simulink model "gm_HDL_pfc_gold_fi_vnl"  (R2024b)
settings: Solver=FixedStepDiscrete  StartTime=0.0  StopTime=.06  RelTol=1e-3
InitFcn:
  | fidelity_pfc_vals;
  | load('C:\Users\angro\Desktop\hil\pfc3ph\matlab\sim\sschdl\pfc_desktop\stateSpaceParameters.mat');
undefined symbols (not defined in the file or in its folder): a, b, c, DiscIntNeverNeededParam, fsw, Gs, s, stateSpaceParameters_1, t_ss, tsw
libraries: simulink x55, hdlmdlgenlib x26, hdlsllib x10, mcbcontrolslib x5, dspsrcs4 x3, slpidlib x2, hdlssclib x2, spsSVPWMGenerator2LevelLib x1, spsPLL3phLib x1
(part 3 of 4)

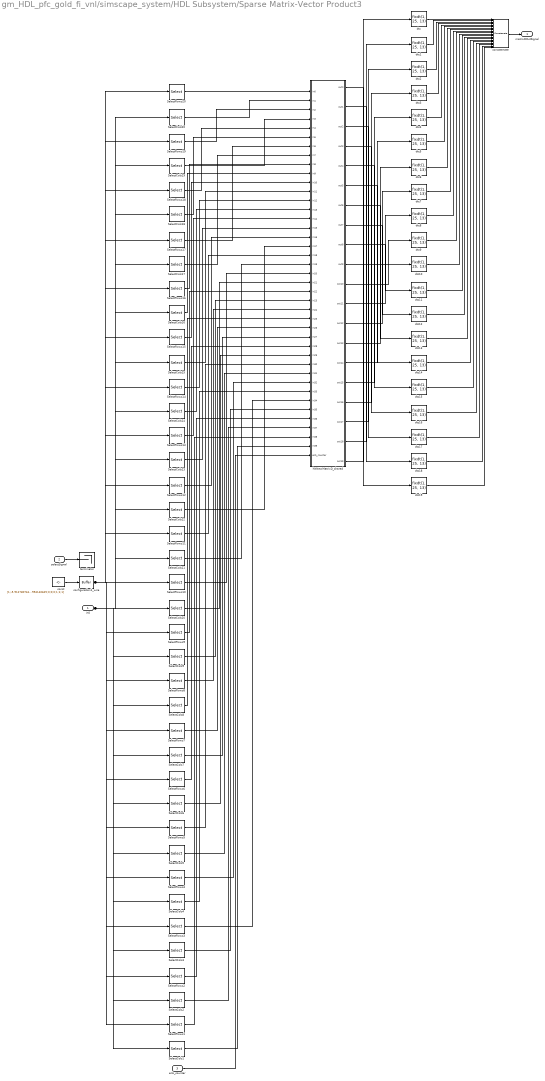
== system gm_HDL_pfc_gold_fi_vnl/simscape_system/HDL Subsystem/Sparse Matrix-Vector Product3 ==
  in0 : Inport  OutDataTypeStr=fixdt(1, 25, 13)  PortDimensions=[10]  SampleTime=1.38600138600139e-08
  selectSignal : Inport  Port=2  OutDataTypeStr=boolean  SampleTime=1.38600138600139e-08
  enb_counter : Inport  Port=3  OutDataTypeStr=fixdt(0, 6, 0)  SampleTime=1.38600138600139e-08
  SelectCols{1..17} (17 alike) : Selector  InputPortWidth=10  IndexOptions=Index vector (dialog)  Indices=double([1 2 3 4 5 6 7])  OutputSizes=double(1)
  SelectCols18 : Selector  InputPortWidth=10  IndexOptions=Index vector (dialog)  Indices=double([1 2 3 4 5 6 9])  OutputSizes=double(1)
  SelectCols19 : Selector  InputPortWidth=10  IndexOptions=Index vector (dialog)  Indices=double([1 2 3 4 5 6 10])  OutputSizes=double(1)
  SelectCols20 : Selector  InputPortWidth=10  IndexOptions=Index vector (dialog)  Indices=double([1 2 3 4 5 6 8])  OutputSizes=double(1)
  SelectRows1 : Selector  InputPortWidth=140  IndexOptions=Index vector (dialog)  Indices=double([1 21 41 61 81 101 121])  OutputSizes=double(1)
  SelectRows10 : Selector  InputPortWidth=140  IndexOptions=Index vector (dialog)  Indices=double([10 30 50 70 90 110 130])  OutputSizes=double(1)
  SelectRows11 : Selector  InputPortWidth=140  IndexOptions=Index vector (dialog)  Indices=double([11 31 51 71 91 111 131])  OutputSizes=double(1)
  SelectRows12 : Selector  InputPortWidth=140  IndexOptions=Index vector (dialog)  Indices=double([12 32 52 72 92 112 132])  OutputSizes=double(1)
  SelectRows13 : Selector  InputPortWidth=140  IndexOptions=Index vector (dialog)  Indices=double([13 33 53 73 93 113 133])  OutputSizes=double(1)
  SelectRows14 : Selector  InputPortWidth=140  IndexOptions=Index vector (dialog)  Indices=double([14 34 54 74 94 114 134])  OutputSizes=double(1)
  SelectRows15 : Selector  InputPortWidth=140  IndexOptions=Index vector (dialog)  Indices=double([15 35 55 75 95 115 135])  OutputSizes=double(1)
  SelectRows16 : Selector  InputPortWidth=140  IndexOptions=Index vector (dialog)  Indices=double([16 36 56 76 96 116 136])  OutputSizes=double(1)
  SelectRows17 : Selector  InputPortWidth=140  IndexOptions=Index vector (dialog)  Indices=double([17 37 57 77 97 117 137])  OutputSizes=double(1)
  SelectRows18 : Selector  InputPortWidth=140  IndexOptions=Index vector (dialog)  Indices=double([18 38 58 78 98 118 139])  OutputSizes=double(1)
  SelectRows19 : Selector  InputPortWidth=140  IndexOptions=Index vector (dialog)  Indices=double([19 39 59 79 99 119 140])  OutputSizes=double(1)
  SelectRows2 : Selector  InputPortWidth=140  IndexOptions=Index vector (dialog)  Indices=double([2 22 42 62 82 102 122])  OutputSizes=double(1)
  SelectRows20 : Selector  InputPortWidth=140  IndexOptions=Index vector (dialog)  Indices=double([20 40 60 80 100 120 138])  OutputSizes=double(1)
  SelectRows3 : Selector  InputPortWidth=140  IndexOptions=Index vector (dialog)  Indices=double([3 23 43 63 83 103 123])  OutputSizes=double(1)
  SelectRows4 : Selector  InputPortWidth=140  IndexOptions=Index vector (dialog)  Indices=double([4 24 44 64 84 104 124])  OutputSizes=double(1)
  SelectRows5 : Selector  InputPortWidth=140  IndexOptions=Index vector (dialog)  Indices=double([5 25 45 65 85 105 125])  OutputSizes=double(1)
  SelectRows6 : Selector  InputPortWidth=140  IndexOptions=Index vector (dialog)  Indices=double([6 26 46 66 86 106 126])  OutputSizes=double(1)
  SelectRows7 : Selector  InputPortWidth=140  IndexOptions=Index vector (dialog)  Indices=double([7 27 47 67 87 107 127])  OutputSizes=double(1)
  SelectRows8 : Selector  InputPortWidth=140  IndexOptions=Index vector (dialog)  Indices=double([8 28 48 68 88 108 128])  OutputSizes=double(1)
  SelectRows9 : Selector  InputPortWidth=140  IndexOptions=Index vector (dialog)  Indices=double([9 29 49 69 89 109 129])  OutputSizes=double(1)
  concatenate : Concatenate  NumInputs=20
  configuration1_wire : hdlmdlgenlib/Buffer
  const : Constant  Value=[1;-5.91278076171875e-05;-0.0030002593994140625;-5.91278076171875e-05;-0.0030002593994140625;-5.91278076171875e-05;-0.0030002593994140625;-5.91278076171875e-05;-0.0030002593994140625;-5.91278076171875e-05;-0.0030002593994140625;-5.91278076171875e-05;-0.0030002593994140625;-0.0059986114501953125;0;0;0;0;0;0;0;-0.499969482421875;25.001499176025390625;-0.499969482421875;-24.998500823974609375;3.0517578125e-05;0.001499176025390625;3.0517578125e-05;0.001499176025390625;3.0517578125e-05;0.001499176025390625;3.0517578125e-05;0.001499176025390625;0.0030002593994140625;0;0;0;0;0;0;0;-0.499969482421875;-24.998500823974609375;-0.499969482421875;25.001499176025390625;3.0517578125e-05;0.001499176025390625;3.0517578125e-05;0.001499176025390625;3.0517578125e-05;0.001499176025390625;3.0517578125e-05;0.001499176025390625;0.0030002593994140625;0;0;0;0;0;0;0;3.0517578125e-05;0.001499176025390625;3.0517578125e-05;0.001499176025390625;-0.499969482421875;25.001499176025390625;3.0517578125e-05;0.001499176025390625;-0.499969482421875;-24.998500823974609375;3.0517578125e-05;0.001499176025390625;0.0030002593994140625;0;0;0;0;0;0;0;3.0517578125e-05;0.001499176025390625;3.0517578125e-05;0.001499176025390625;3.0517578125e-05;0.001499176025390625;-0.499969482421875;25.001499176025390625;3.0517578125e-05;0.001499176025390625;-0.499969482421875;-24.998500823974609375;0.0030002593994140625;0;0;0;0;0;0;0;3.0517578125e-05;0.001499176025390625;3.0517578125e-05;0.001499176025390625;-0.499969482421875;-24.998500823974609375;3.0517578125e-05;0.001499176025390625;-0.499969482421875;25.001499176025390625;3.0517578125e-05;0.001499176025390625;0.0030002593994140625;0;0;0;0;0;0;0;3.0517578125e-05;0.001499176025390625;3.0517578125e-05;0.001499176025390625;3.0517578125e-05;0.001499176025390625;-0.499969482421875;-24.998500823974609375;3.0517578125e-05;0.001499176025390625;-0.499969482421875;25.001499176025390625;0.0030002593994140625;0;0;0;1;1;1]  OutDataTypeStr=fixdt(1, 25, 19)  SampleTime=1.38600138600139e-08
  dtc{,1..19} (20 alike) : DataTypeConversion  OutDataTypeStr=fixdt(1, 25, 13)  RndMeth=Nearest  SampleTime=1.38600138600139e-08  SaturateOnIntegerOverflow=off
  hNNewMatrixD_shared : Subsystem
  terminator : Terminator
  matrixDOutSignal : Outport  OutDataTypeStr=fixdt(1, 25, 13)  PortDimensions=[20]  SampleTime=1.38600138600139e-08
  wires:
  concatenate/1 -> matrixDOutSignal/1
  dtc19/1 -> concatenate/20
  dtc18/1 -> concatenate/19
  dtc17/1 -> concatenate/18
  dtc16/1 -> concatenate/17
  dtc15/1 -> concatenate/16
  dtc14/1 -> concatenate/15
  dtc13/1 -> concatenate/14
  dtc12/1 -> concatenate/13
  dtc11/1 -> concatenate/12
  dtc10/1 -> concatenate/11
  dtc9/1 -> concatenate/10
  dtc8/1 -> concatenate/9
  dtc6/1 -> concatenate/7
  dtc5/1 -> concatenate/6
  dtc4/1 -> concatenate/5
  dtc3/1 -> concatenate/4
  dtc2/1 -> concatenate/3
  dtc1/1 -> concatenate/2
  dtc/1 -> concatenate/1
  hNNewMatrixD_shared/20(out19) -> dtc/1
  hNNewMatrixD_shared/14(out13) -> dtc6/1
  hNNewMatrixD_shared/13(out12) -> dtc7/1
  hNNewMatrixD_shared/12(out11) -> dtc8/1
  hNNewMatrixD_shared/11(out10) -> dtc9/1
  hNNewMatrixD_shared/10(out9) -> dtc10/1
  hNNewMatrixD_shared/5(out4) -> dtc15/1
  SelectCols1/1 -> hNNewMatrixD_shared/40(in39)
  hNNewMatrixD_shared/6(out5) -> dtc14/1
  SelectRows2/1 -> hNNewMatrixD_shared/37(in36)
  hNNewMatrixD_shared/15(out14) -> dtc5/1
  SelectCols3/1 -> hNNewMatrixD_shared/36(in35)
  hNNewMatrixD_shared/3(out2) -> dtc17/1
  SelectRows3/1 -> hNNewMatrixD_shared/35(in34)
  SelectRows4/1 -> hNNewMatrixD_shared/33(in32)
  hNNewMatrixD_shared/9(out8) -> dtc11/1
  SelectCols5/1 -> hNNewMatrixD_shared/32(in31)
  SelectRows5/1 -> hNNewMatrixD_shared/31(in30)
  SelectRows6/1 -> hNNewMatrixD_shared/29(in28)
  SelectCols8/1 -> hNNewMatrixD_shared/26(in25)
  SelectCols4/1 -> hNNewMatrixD_shared/34(in33)
  hNNewMatrixD_shared/4(out3) -> dtc16/1
  SelectRows8/1 -> hNNewMatrixD_shared/25(in24)
  SelectCols9/1 -> hNNewMatrixD_shared/24(in23)
  SelectRows1/1 -> hNNewMatrixD_shared/39(in38)
  SelectRows9/1 -> hNNewMatrixD_shared/23(in22)
  dtc7/1 -> concatenate/8
  hNNewMatrixD_shared/19(out18) -> dtc1/1
  SelectRows10/1 -> hNNewMatrixD_shared/21(in20)
  SelectCols2/1 -> hNNewMatrixD_shared/38(in37)
  hNNewMatrixD_shared/2(out1) -> dtc18/1
  SelectCols11/1 -> hNNewMatrixD_shared/20(in19)
  SelectRows7/1 -> hNNewMatrixD_shared/27(in26)
  SelectCols7/1 -> hNNewMatrixD_shared/28(in27)
  SelectRows11/1 -> hNNewMatrixD_shared/19(in18)
  SelectCols12/1 -> hNNewMatrixD_shared/18(in17)
  hNNewMatrixD_shared/18(out17) -> dtc2/1
  SelectRows12/1 -> hNNewMatrixD_shared/17(in16)
  SelectRows13/1 -> hNNewMatrixD_shared/15(in14)
  SelectCols14/1 -> hNNewMatrixD_shared/14(in13)
  hNNewMatrixD_shared/17(out16) -> dtc3/1
  SelectRows14/1 -> hNNewMatrixD_shared/13(in12)
  SelectCols6/1 -> hNNewMatrixD_shared/30(in29)
  hNNewMatrixD_shared/1(out0) -> dtc19/1
  SelectCols15/1 -> hNNewMatrixD_shared/12(in11)
  SelectRows15/1 -> hNNewMatrixD_shared/11(in10)
  SelectCols16/1 -> hNNewMatrixD_shared/10(in9)
  SelectCols13/1 -> hNNewMatrixD_shared/16(in15)
  hNNewMatrixD_shared/16(out15) -> dtc4/1
  SelectRows16/1 -> hNNewMatrixD_shared/9(in8)
  SelectCols17/1 -> hNNewMatrixD_shared/8(in7)
  SelectRows17/1 -> hNNewMatrixD_shared/7(in6)
  enb_counter/1 -> hNNewMatrixD_shared/41(enb_counter)
  SelectCols18/1 -> hNNewMatrixD_shared/6(in5)
  SelectRows19/1 -> hNNewMatrixD_shared/3(in2)
  hNNewMatrixD_shared/7(out6) -> dtc13/1
  SelectCols20/1 -> hNNewMatrixD_shared/2(in1)
  in0/1 -> SelectCols4/1, SelectCols1/1, SelectCols2/1, SelectCols5/1, SelectCols3/1, SelectCols8/1, SelectCols6/1, SelectCols7/1, SelectCols9/1, SelectCols10/1, SelectCols11/1, SelectCols12/1, SelectCols16/1, SelectCols13/1, SelectCols14/1, SelectCols15/1, SelectCols17/1, SelectCols18/1, SelectCols19/1, SelectCols20/1
  hNNewMatrixD_shared/8(out7) -> dtc12/1
  configuration1_wire/1 -> SelectRows1/1, SelectRows12/1, SelectRows5/1, SelectRows14/1, SelectRows3/1, SelectRows15/1, SelectRows2/1, SelectRows6/1, SelectRows4/1, SelectRows10/1, SelectRows8/1, SelectRows7/1, SelectRows9/1, SelectRows11/1, SelectRows13/1, SelectRows16/1, SelectRows19/1, SelectRows17/1, SelectRows18/1, SelectRows20/1
  const/1 -> configuration1_wire/1
  SelectCols19/1 -> hNNewMatrixD_shared/4(in3)
  SelectCols10/1 -> hNNewMatrixD_shared/22(in21)
  SelectRows20/1 -> hNNewMatrixD_shared/1(in0)
  selectSignal/1 -> terminator/1
  SelectRows18/1 -> hNNewMatrixD_shared/5(in4)

== system gm_HDL_pfc_gold_fi_vnl/simscape_system/HDL Subsystem/streaming_partition_streamed ==
  in0 : Inport  OutDataTypeStr=fixdt(1, 25, 13)  PortDimensions=[7]  SampleTime=1.38600138600139e-08
  in1 : Inport  Port=2  OutDataTypeStr=fixdt(1, 25, 13)  PortDimensions=[7]  SampleTime=1.38600138600139e-08
  enb_counter : Inport  Port=3  OutDataTypeStr=fixdt(0, 6, 0)  SampleTime=1.38600138600139e-08
  Serializer_Subnetwork : Subsystem
  Serializer_Subnetwork1 : Subsystem
  counter : Subsystem
  delayInSignal_bypass : Subsystem
  delayMatch : Delay  DelayLength=double(1)  InitialCondition=0  SampleTime=1.38600138600139e-08
  delayMatch1 : Delay  DelayLength=double(1)  InitialCondition=0  SampleTime=1.38600138600139e-08
  dtc : hdlmdlgenlib/Buffer
  enb_counter_eq_20 : simulink/Logic and Bit Operations/Compare To Constant  relop===  const=double(20)  OutDataTypeStr=boolean
  enb_counter_ge_13 : simulink/Logic and Bit Operations/Compare To Constant  relop=>=  const=double(13)  OutDataTypeStr=boolean
  enb_counter_ge_13_and_enb_counter_le_19 : Logic  AllPortsSameDT=off  OutDataTypeStr=boolean  SampleTime=1.38600138600139e-08
  enb_counter_ge_14 : simulink/Logic and Bit Operations/Compare To Constant  relop=>=  const=double(14)  OutDataTypeStr=boolean
  enb_counter_ge_14_and_enb_counter_le_19 : Logic  AllPortsSameDT=off  OutDataTypeStr=boolean  SampleTime=1.38600138600139e-08
  enb_counter_le_19 : simulink/Logic and Bit Operations/Compare To Constant  relop=<=  const=double(19)  OutDataTypeStr=boolean
  enb_counter_le_191 : simulink/Logic and Bit Operations/Compare To Constant  relop=<=  const=double(19)  OutDataTypeStr=boolean
  sumStateEqnComp : Sum  OutDataTypeStr=fixdt(1, 25, 13)  SampleTime=1.38600138600139e-08
  t : Mux  Inputs=2
  tappedDelay : Subsystem
  out0 : Outport  OutDataTypeStr=fixdt(1, 25, 13)  PortDimensions=[7]  SampleTime=1.38600138600139e-08
  wires:
  delayInSignal_bypass/1(out0) -> t/2
  tappedDelay/1(out0) -> t/1
  dtc/1 -> delayInSignal_bypass/1(in0), tappedDelay/1(in0)
  enb_counter_eq_20/1 -> delayInSignal_bypass/2(in1)
  sumStateEqnComp/1 -> dtc/1
  Serializer_Subnetwork1/1(out0) -> sumStateEqnComp/2
  delayMatch/1 -> sumStateEqnComp/1
  t/1 -> out0/1
  delayMatch1/1 -> Serializer_Subnetwork1/2(in1)
  in1/1 -> Serializer_Subnetwork1/1(in0)
  Serializer_Subnetwork/1(out0) -> delayMatch/1
  counter/1(out0) -> Serializer_Subnetwork/2(in1), delayMatch1/1
  enb_counter_ge_13_and_enb_counter_le_19/1 -> counter/Enable
  enb_counter_ge_14_and_enb_counter_le_19/1 -> tappedDelay/Enable
  enb_counter_le_19/1 -> enb_counter_ge_13_and_enb_counter_le_19/2
  enb_counter_le_191/1 -> enb_counter_ge_14_and_enb_counter_le_19/2
  in0/1 -> Serializer_Subnetwork/1(in0)
  enb_counter_ge_14/1 -> enb_counter_ge_14_and_enb_counter_le_19/1
  enb_counter/1 -> enb_counter_ge_13/1, enb_counter_eq_20/1, enb_counter_le_191/1, enb_counter_le_19/1, enb_counter_ge_14/1
  enb_counter_ge_13/1 -> enb_counter_ge_13_and_enb_counter_le_19/1

== system gm_HDL_pfc_gold_fi_vnl/simscape_system/HDL Subsystem/streaming_partition_streamed1 ==
  in0 : Inport  OutDataTypeStr=fixdt(1, 25, 13)  PortDimensions=[7]  SampleTime=1.38600138600139e-08
  in1 : Inport  Port=2  OutDataTypeStr=boolean  SampleTime=1.38600138600139e-08
  in2 : Inport  Port=3  OutDataTypeStr=fixdt(1, 25, 13)  PortDimensions=[7]  SampleTime=1.38600138600139e-08
  enb_counter : Inport  Port=4  OutDataTypeStr=fixdt(0, 6, 0)  SampleTime=1.38600138600139e-08
  Serializer_Subnetwork : Subsystem
  Serializer_Subnetwork1 : Subsystem
  State_switch : Switch  Criteria=u2 ~= 0  Threshold=double(0)  OutDataTypeStr=fixdt(1, 25, 13)  SampleTime=1.38600138600139e-08  SaturateOnIntegerOverflow=off  InputSameDT=off
  counter : Subsystem
  delayOutSignal_bypass : Subsystem
  enb_counter_eq_6 : simulink/Logic and Bit Operations/Compare To Constant  relop===  const=double(6)  OutDataTypeStr=boolean
  enb_counter_le_5 : simulink/Logic and Bit Operations/Compare To Constant  relop=<=  const=double(5)  OutDataTypeStr=boolean
  enb_counter_le_6 : simulink/Logic and Bit Operations/Compare To Constant  relop=<=  const=double(6)  OutDataTypeStr=boolean
  t : Mux  Inputs=2
  tappedDelay : Subsystem
  out0 : Outport  OutDataTypeStr=fixdt(1, 25, 13)  PortDimensions=[7]  SampleTime=1.38600138600139e-08
  wires:
  t/1 -> out0/1
  delayOutSignal_bypass/1(out0) -> t/2
  enb_counter_le_5/1 -> tappedDelay/Enable
  Serializer_Subnetwork1/1(out0) -> State_switch/3
  in1/1 -> State_switch/2
  in2/1 -> Serializer_Subnetwork1/1(in0)
  in0/1 -> Serializer_Subnetwork/1(in0)
  tappedDelay/1(out0) -> t/1
  counter/1(out0) -> Serializer_Subnetwork1/2(in1), Serializer_Subnetwork/2(in1)
  State_switch/1 -> delayOutSignal_bypass/1(in0), tappedDelay/1(in0)
  enb_counter_eq_6/1 -> delayOutSignal_bypass/2(in1)
  enb_counter_le_6/1 -> counter/Enable
  Serializer_Subnetwork/1(out0) -> State_switch/1
  enb_counter/1 -> enb_counter_eq_6/1, enb_counter_le_6/1, enb_counter_le_5/1

== system gm_HDL_pfc_gold_fi_vnl/simscape_system_vnl/HDL Subsystem/HDL Algorithm ==
  In1 : Inport
  Delay1 : Delay  DelayLength=1
  Delay2 : Delay
  Output : Subsystem
  Sel : Constant  Value=0  OutDataTypeStr=uint32  SampleTime=-1
  State Delay : Delay  DelayLength=1  InitialCondition=single(stateSpaceParameters_1.X0)
  State Switch : Switch  Criteria=u2 ~= 0  SaturateOnIntegerOverflow=off  InputSameDT=off
  State Update : Subsystem
  Valid Out : Constant  OutDataTypeStr=boolean  SampleTime=4.395604395604395e-07
  X0 : Constant  Value=single(stateSpaceParameters_1.X0)  SampleTime=4.395604395604395e-07
  Out1 : Outport  VectorParamsAs1DForOutWhenUnconnected=off
  wires:
  In1/1 -> State Update/1(In1), Delay1/1
  State Switch/1 -> State Update/2(State), Output/2(State)
  Output/1(Out1) -> Out1/1
  X0/1 -> State Switch/3
  Delay2/1 -> State Switch/2
  State Delay/1 -> State Switch/1
  Valid Out/1 -> Delay2/1
  State Update/1(State Out) -> State Delay/1
  Sel/1 -> State Update/3(Sel), Output/3(Sel)
  Delay1/1 -> Output/1(In1)

== system gm_HDL_pfc_gold_fi_vnl/Subsystem1/ctrl_pwm/transforms/Claro-Parl Transform ==
  a : Inport
  b : Inport  Port=2
  wt : Inport  Port=3
  Clarke Transform : mcbcontrolslib/Clarke Transform  VariantControl=Variant2  PhaseInput=Two inputs  EnPowerInv=off
  Cos : Trigonometry  Operator=cos
  Park Transform : mcbcontrolslib/Park Transform  PhaseInput=Two inputs  AxisAlignment=D-axis  ThetaInput=Sine and Cosine electrical position  AngleInput=Per-unit  N_points=1024
  Sin : Trigonometry
  d : Outport
  q : Outport  Port=2
  wires:
  Clarke Transform/2 -> Park Transform/2  "Vbet_sourc"
  b/1 -> Clarke Transform/2
  Park Transform/2 -> q/1
  Park Transform/1 -> d/1
  Clarke Transform/1 -> Park Transform/1  "Valp_sourc"
  wt/1 -> Cos/1, Sin/1
  a/1 -> Clarke Transform/1
  Sin/1 -> Park Transform/3
  Cos/1 -> Park Transform/4

== system gm_HDL_pfc_gold_fi_vnl/Subsystem1/ctrl_pwm/transforms/Claro-Parl Transform1 ==
  a : Inport
  b : Inport  Port=2
  wt : Inport  Port=3
  Clarke Transform : mcbcontrolslib/Clarke Transform  VariantControl=Variant2  PhaseInput=Two inputs  EnPowerInv=off
  Cos : Trigonometry  Operator=cos
  Park Transform : mcbcontrolslib/Park Transform  PhaseInput=Two inputs  AxisAlignment=D-axis  ThetaInput=Sine and Cosine electrical position  AngleInput=Per-unit  N_points=1024
  Sin : Trigonometry
  d : Outport
  q : Outport  Port=2
  wires:
  Clarke Transform/2 -> Park Transform/2  "Ibet_sourc"
  b/1 -> Clarke Transform/2
  Park Transform/2 -> q/1
  Park Transform/1 -> d/1
  Clarke Transform/1 -> Park Transform/1  "Ialp_sourc"
  wt/1 -> Cos/1, Sin/1
  a/1 -> Clarke Transform/1
  Sin/1 -> Park Transform/3
  Cos/1 -> Park Transform/4

== system gm_HDL_pfc_gold_fi_vnl/simscape_system/FET_CTRL/crp_temp_streamed/Discrete-Time Integrator_u_sat_bypass ==
  in0 : Inport  OutDataTypeStr=fixdt(1, 18, 8)  PortDimensions=[5]  SampleTime=1.38600138600139e-08
  in1 : Inport  Port=2  OutDataTypeStr=boolean  SampleTime=1.38600138600139e-08
  Discrete-Time Integrator_u_sat_enb : Switch  Criteria=u2 ~= 0  Threshold=double(0)  OutDataTypeStr=fixdt(1, 18, 8)  SampleTime=1.38600138600139e-08  SaturateOnIntegerOverflow=off  InputSameDT=off
  Discrete-Time Integrator_u_sat_state : Delay  DelayLength=double(1)  InitialCondition=0  SampleTime=1.38600138600139e-08
  out0 : Outport  OutDataTypeStr=fixdt(1, 18, 8)  PortDimensions=[5]  SampleTime=1.38600138600139e-08
  wires:
  Discrete-Time Integrator_u_sat_state/1 -> Discrete-Time Integrator_u_sat_enb/3
  in1/1 -> Discrete-Time Integrator_u_sat_enb/2
  in0/1 -> Discrete-Time Integrator_u_sat_enb/1
  Discrete-Time Integrator_u_sat_enb/1 -> out0/1, Discrete-Time Integrator_u_sat_state/1

== system gm_HDL_pfc_gold_fi_vnl/simscape_system/FET_CTRL/crp_temp_streamed/Discrete-Time Integrator_u_sat_bypass1 ==
  in0 : Inport  OutDataTypeStr=fixdt(1, 18, 8)  SampleTime=1.38600138600139e-08
  in1 : Inport  Port=2  OutDataTypeStr=boolean  SampleTime=1.38600138600139e-08
  Discrete-Time Integrator_u_sat_enb : Switch  Criteria=u2 ~= 0  Threshold=double(0)  OutDataTypeStr=fixdt(1, 18, 8)  SampleTime=1.38600138600139e-08  SaturateOnIntegerOverflow=off  InputSameDT=off
  Discrete-Time Integrator_u_sat_state : Delay  DelayLength=double(1)  InitialCondition=0  SampleTime=1.38600138600139e-08
  out0 : Outport  OutDataTypeStr=fixdt(1, 18, 8)  SampleTime=1.38600138600139e-08
  wires:
  Discrete-Time Integrator_u_sat_enb/1 -> out0/1, Discrete-Time Integrator_u_sat_state/1
  Discrete-Time Integrator_u_sat_state/1 -> Discrete-Time Integrator_u_sat_enb/3
  in1/1 -> Discrete-Time Integrator_u_sat_enb/2
  in0/1 -> Discrete-Time Integrator_u_sat_enb/1

== system gm_HDL_pfc_gold_fi_vnl/simscape_system/FET_CTRL/crp_temp_streamed/Serializer_Subnetwork ==
  in0 : Inport  OutDataTypeStr=fixdt(1, 18, 8)  PortDimensions=[6]  SampleTime=1.38600138600139e-08
  in1 : Inport  Port=2  OutDataTypeStr=fixdt(0, 3, 0)  SampleTime=1.38600138600139e-08
  ratechange_splitcomp : Demux  Outputs=6
  splitcomp_multiport : MultiPortSwitch  DataPortOrder=Zero-based contiguous  Inputs=6  DiagnosticForDefault=None  zeroidx=on  OutDataTypeStr=fixdt(1, 18, 8)  SampleTime=1.38600138600139e-08  SaturateOnIntegerOverflow=off  InputSameDT=off
  out0 : Outport  OutDataTypeStr=fixdt(1, 18, 8)  SampleTime=1.38600138600139e-08
  wires:
  splitcomp_multiport/1 -> out0/1
  ratechange_splitcomp/6 -> splitcomp_multiport/7
  ratechange_splitcomp/5 -> splitcomp_multiport/6
  ratechange_splitcomp/4 -> splitcomp_multiport/5
  ratechange_splitcomp/3 -> splitcomp_multiport/4
  ratechange_splitcomp/2 -> splitcomp_multiport/3
  ratechange_splitcomp/1 -> splitcomp_multiport/2
  in1/1 -> splitcomp_multiport/1
  in0/1 -> ratechange_splitcomp/1

== system gm_HDL_pfc_gold_fi_vnl/simscape_system/FET_CTRL/crp_temp_streamed/Serializer_Subnetwork1 ==
  in0 : Inport  OutDataTypeStr=boolean  PortDimensions=[6]  SampleTime=1.38600138600139e-08
  in1 : Inport  Port=2  OutDataTypeStr=fixdt(0, 3, 0)  SampleTime=1.38600138600139e-08
  ratechange_splitcomp : Demux  Outputs=6
  splitcomp_multiport : MultiPortSwitch  DataPortOrder=Zero-based contiguous  Inputs=6  DiagnosticForDefault=None  zeroidx=on  SampleTime=1.38600138600139e-08  SaturateOnIntegerOverflow=off  InputSameDT=off
  out0 : Outport  OutDataTypeStr=boolean  SampleTime=1.38600138600139e-08
  wires:
  splitcomp_multiport/1 -> out0/1
  ratechange_splitcomp/4 -> splitcomp_multiport/5
  ratechange_splitcomp/3 -> splitcomp_multiport/4
  ratechange_splitcomp/2 -> splitcomp_multiport/3
  ratechange_splitcomp/1 -> splitcomp_multiport/2
  in1/1 -> splitcomp_multiport/1
  in0/1 -> ratechange_splitcomp/1
  ratechange_splitcomp/6 -> splitcomp_multiport/7
  ratechange_splitcomp/5 -> splitcomp_multiport/6

== system gm_HDL_pfc_gold_fi_vnl/simscape_system/FET_CTRL/crp_temp_streamed/Serializer_Subnetwork2 ==
  in0 : Inport  OutDataTypeStr=fixdt(1, 18, 6)  PortDimensions=[6]  SampleTime=1.38600138600139e-08
  in1 : Inport  Port=2  OutDataTypeStr=fixdt(0, 3, 0)  SampleTime=1.38600138600139e-08
  ratechange_splitcomp : Demux  Outputs=6
  splitcomp_multiport : MultiPortSwitch  DataPortOrder=Zero-based contiguous  Inputs=6  DiagnosticForDefault=None  zeroidx=on  OutDataTypeStr=fixdt(1, 18, 6)  SampleTime=1.38600138600139e-08  SaturateOnIntegerOverflow=off  InputSameDT=off
  out0 : Outport  OutDataTypeStr=fixdt(1, 18, 6)  SampleTime=1.38600138600139e-08
  wires:
  splitcomp_multiport/1 -> out0/1
  ratechange_splitcomp/5 -> splitcomp_multiport/6
  ratechange_splitcomp/4 -> splitcomp_multiport/5
  ratechange_splitcomp/3 -> splitcomp_multiport/4
  ratechange_splitcomp/2 -> splitcomp_multiport/3
  ratechange_splitcomp/1 -> splitcomp_multiport/2
  in1/1 -> splitcomp_multiport/1
  ratechange_splitcomp/6 -> splitcomp_multiport/7
  in0/1 -> ratechange_splitcomp/1

== system gm_HDL_pfc_gold_fi_vnl/simscape_system/FET_CTRL/crp_temp_streamed/Serializer_Subnetwork3 ==
  in0 : Inport  OutDataTypeStr=fixdt(1, 18, 6)  PortDimensions=[6]  SampleTime=1.38600138600139e-08
  in1 : Inport  Port=2  OutDataTypeStr=fixdt(0, 3, 0)  SampleTime=1.38600138600139e-08
  ratechange_splitcomp : Demux  Outputs=6
  splitcomp_multiport : MultiPortSwitch  DataPortOrder=Zero-based contiguous  Inputs=6  DiagnosticForDefault=None  zeroidx=on  OutDataTypeStr=fixdt(1, 18, 6)  SampleTime=1.38600138600139e-08  SaturateOnIntegerOverflow=off  InputSameDT=off
  out0 : Outport  OutDataTypeStr=fixdt(1, 18, 6)  SampleTime=1.38600138600139e-08
  wires:
  splitcomp_multiport/1 -> out0/1
  ratechange_splitcomp/4 -> splitcomp_multiport/5
  ratechange_splitcomp/3 -> splitcomp_multiport/4
  ratechange_splitcomp/2 -> splitcomp_multiport/3
  ratechange_splitcomp/1 -> splitcomp_multiport/2
  in1/1 -> splitcomp_multiport/1
  in0/1 -> ratechange_splitcomp/1
  ratechange_splitcomp/6 -> splitcomp_multiport/7
  ratechange_splitcomp/5 -> splitcomp_multiport/6

== system gm_HDL_pfc_gold_fi_vnl/simscape_system/FET_CTRL/crp_temp_streamed/buffSig_bypass ==
  in0 : Inport  OutDataTypeStr=fixdt(1, 18, 8)  PortDimensions=[5]  SampleTime=1.38600138600139e-08
  in1 : Inport  Port=2  OutDataTypeStr=boolean  SampleTime=1.38600138600139e-08
  buffSig_enb : Switch  Criteria=u2 ~= 0  Threshold=double(0)  OutDataTypeStr=fixdt(1, 18, 8)  SampleTime=1.38600138600139e-08  SaturateOnIntegerOverflow=off  InputSameDT=off
  buffSig_state : Delay  DelayLength=double(1)  InitialCondition=0  SampleTime=1.38600138600139e-08
  out0 : Outport  OutDataTypeStr=fixdt(1, 18, 8)  PortDimensions=[5]  SampleTime=1.38600138600139e-08
  wires:
  buffSig_enb/1 -> out0/1, buffSig_state/1
  buffSig_state/1 -> buffSig_enb/3
  in1/1 -> buffSig_enb/2
  in0/1 -> buffSig_enb/1

== system gm_HDL_pfc_gold_fi_vnl/simscape_system/FET_CTRL/crp_temp_streamed/buffSig_bypass1 ==
  in0 : Inport  OutDataTypeStr=fixdt(1, 18, 8)  SampleTime=1.38600138600139e-08
  in1 : Inport  Port=2  OutDataTypeStr=boolean  SampleTime=1.38600138600139e-08
  buffSig_enb : Switch  Criteria=u2 ~= 0  Threshold=double(0)  OutDataTypeStr=fixdt(1, 18, 8)  SampleTime=1.38600138600139e-08  SaturateOnIntegerOverflow=off  InputSameDT=off
  buffSig_state : Delay  DelayLength=double(1)  InitialCondition=0  SampleTime=1.38600138600139e-08
  out0 : Outport  OutDataTypeStr=fixdt(1, 18, 8)  SampleTime=1.38600138600139e-08
  wires:
  buffSig_enb/1 -> out0/1, buffSig_state/1
  buffSig_state/1 -> buffSig_enb/3
  in1/1 -> buffSig_enb/2
  in0/1 -> buffSig_enb/1

== system gm_HDL_pfc_gold_fi_vnl/simscape_system/FET_CTRL/crp_temp_streamed/counter ==
  globalSchedule : EnablePort  OutDataTypeStr=boolean
  ctr_0_5 : hdlsllib/Sources/HDL Counter  CountType=Count limited  CountInit=double(0)  CountStep=double(1)  CountMax=double(5)  CountFromType=Initial value  CountFrom=double(0)  CountResetPort=off  CountLoadPort=off  CountEnbPort=off  CountDirPort=off  CountHitOutputPort=off  CountDataType=Unsigned  CountWordLen=3  CountFracLen=0  CountSampTime=1.38600138600139e-08
  out0 : Outport  OutDataTypeStr=fixdt(0, 3, 0)  SampleTime=1.38600138600139e-08  InitialOutput=0
  wires:
  ctr_0_5/1 -> out0/1

== system gm_HDL_pfc_gold_fi_vnl/simscape_system/FET_CTRL/crp_temp_streamed/tappedDelay ==
  in0 : Inport  OutDataTypeStr=fixdt(1, 18, 8)  SampleTime=1.38600138600139e-08
  globalSchedule : EnablePort  OutDataTypeStr=boolean
  StateControl : StateControl  StateControl=Synchronous
  tapped_delay : simulink/Discrete/Tapped Delay  vinit=0  samptime=-1  NumDelays=double(5)  DelayOrder=Oldest  includeCurrent=off
  out0 : Outport  OutDataTypeStr=fixdt(1, 18, 8)  PortDimensions=[5]  SampleTime=1.38600138600139e-08  InitialOutput=0
  wires:
  tapped_delay/1 -> out0/1
  in0/1 -> tapped_delay/1

== system gm_HDL_pfc_gold_fi_vnl/simscape_system/FET_CTRL/crp_temp_streamed/tappedDelay1 ==
  in0 : Inport  OutDataTypeStr=fixdt(1, 18, 8)  SampleTime=1.38600138600139e-08
  globalSchedule : EnablePort  OutDataTypeStr=boolean
  StateControl : StateControl  StateControl=Synchronous
  tapped_delay : simulink/Discrete/Tapped Delay  vinit=0  samptime=-1  NumDelays=double(5)  DelayOrder=Oldest  includeCurrent=off
  out0 : Outport  OutDataTypeStr=fixdt(1, 18, 8)  PortDimensions=[5]  SampleTime=1.38600138600139e-08  InitialOutput=0
  wires:
  tapped_delay/1 -> out0/1
  in0/1 -> tapped_delay/1

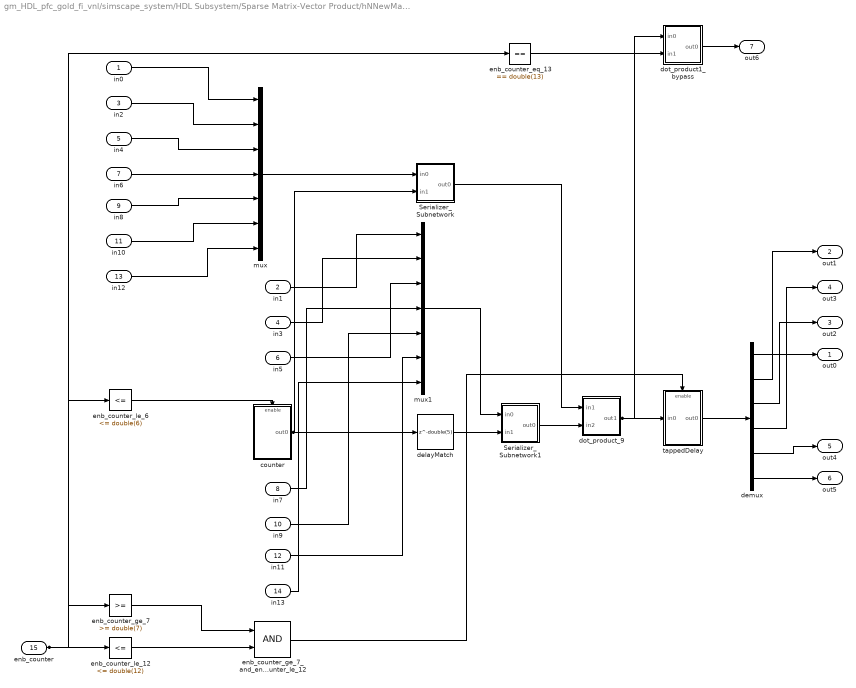
== system gm_HDL_pfc_gold_fi_vnl/simscape_system/HDL Subsystem/Sparse Matrix-Vector Product/hNNewMatrixB_shared ==
  in0 : Inport  OutDataTypeStr=fixdt(1, 25, 31)  PortDimensions=[9]  SampleTime=1.38600138600139e-08
  in1 : Inport  Port=2  OutDataTypeStr=fixdt(1, 25, 13)  PortDimensions=[9]  SampleTime=1.38600138600139e-08
  in2 : Inport  Port=3  OutDataTypeStr=fixdt(1, 25, 31)  PortDimensions=[9]  SampleTime=1.38600138600139e-08
  in3 : Inport  Port=4  OutDataTypeStr=fixdt(1, 25, 13)  PortDimensions=[9]  SampleTime=1.38600138600139e-08
  in4 : Inport  Port=5  OutDataTypeStr=fixdt(1, 25, 31)  PortDimensions=[9]  SampleTime=1.38600138600139e-08
  in5 : Inport  Port=6  OutDataTypeStr=fixdt(1, 25, 13)  PortDimensions=[9]  SampleTime=1.38600138600139e-08
  in6 : Inport  Port=7  OutDataTypeStr=fixdt(1, 25, 31)  PortDimensions=[9]  SampleTime=1.38600138600139e-08
  in7 : Inport  Port=8  OutDataTypeStr=fixdt(1, 25, 13)  PortDimensions=[9]  SampleTime=1.38600138600139e-08
  in8 : Inport  Port=9  OutDataTypeStr=fixdt(1, 25, 31)  PortDimensions=[9]  SampleTime=1.38600138600139e-08
  in9 : Inport  Port=10  OutDataTypeStr=fixdt(1, 25, 13)  PortDimensions=[9]  SampleTime=1.38600138600139e-08
  in10 : Inport  Port=11  OutDataTypeStr=fixdt(1, 25, 31)  PortDimensions=[9]  SampleTime=1.38600138600139e-08
  in11 : Inport  Port=12  OutDataTypeStr=fixdt(1, 25, 13)  PortDimensions=[9]  SampleTime=1.38600138600139e-08
  in12 : Inport  Port=13  OutDataTypeStr=fixdt(1, 25, 31)  PortDimensions=[9]  SampleTime=1.38600138600139e-08
  in13 : Inport  Port=14  OutDataTypeStr=fixdt(1, 25, 13)  PortDimensions=[9]  SampleTime=1.38600138600139e-08
  enb_counter : Inport  Port=15  OutDataTypeStr=fixdt(0, 6, 0)  SampleTime=1.38600138600139e-08
  Serializer_Subnetwork : Subsystem
  Serializer_Subnetwork1 : Subsystem
  counter : Subsystem
  delayMatch : Delay  DelayLength=double(5)  InitialCondition=0  SampleTime=1.38600138600139e-08
  demux : Demux  Outputs=6
  dot_product1_bypass : Subsystem
  dot_product_9 : Subsystem
  enb_counter_eq_13 : simulink/Logic and Bit Operations/Compare To Constant  relop===  const=double(13)  OutDataTypeStr=boolean
  enb_counter_ge_7 : simulink/Logic and Bit Operations/Compare To Constant  relop=>=  const=double(7)  OutDataTypeStr=boolean
  enb_counter_ge_7_and_enb_counter_le_12 : Logic  AllPortsSameDT=off  OutDataTypeStr=boolean  SampleTime=1.38600138600139e-08
  enb_counter_le_12 : simulink/Logic and Bit Operations/Compare To Constant  relop=<=  const=double(12)  OutDataTypeStr=boolean
  enb_counter_le_6 : simulink/Logic and Bit Operations/Compare To Constant  relop=<=  const=double(6)  OutDataTypeStr=boolean
  mux : Mux  Inputs=7
  mux1 : Mux  Inputs=7
  tappedDelay : Subsystem
  out0 : Outport  OutDataTypeStr=fixdt(1, 50, 44)  SampleTime=1.38600138600139e-08
  out1 : Outport  Port=2  OutDataTypeStr=fixdt(1, 50, 44)  SampleTime=1.38600138600139e-08
  out2 : Outport  Port=3  OutDataTypeStr=fixdt(1, 50, 44)  SampleTime=1.38600138600139e-08
  out3 : Outport  Port=4  OutDataTypeStr=fixdt(1, 50, 44)  SampleTime=1.38600138600139e-08
  out4 : Outport  Port=5  OutDataTypeStr=fixdt(1, 50, 44)  SampleTime=1.38600138600139e-08
  out5 : Outport  Port=6  OutDataTypeStr=fixdt(1, 50, 44)  SampleTime=1.38600138600139e-08
  out6 : Outport  Port=7  OutDataTypeStr=fixdt(1, 50, 44)  SampleTime=1.38600138600139e-08
  wires:
  demux/1 -> out0/1
  demux/2 -> out1/1
  tappedDelay/1(out0) -> demux/1
  dot_product_9/1(out1) -> dot_product1_bypass/1(in0), tappedDelay/1(in0)
  Serializer_Subnetwork1/1(out0) -> dot_product_9/2(in2)
  enb_counter_eq_13/1 -> dot_product1_bypass/2(in1)
  mux1/1 -> Serializer_Subnetwork1/1(in0)
  Serializer_Subnetwork/1(out0) -> dot_product_9/1(in1)
  dot_product1_bypass/1(out0) -> out6/1
  enb_counter_ge_7_and_enb_counter_le_12/1 -> tappedDelay/Enable
  in13/1 -> mux1/7
  demux/5 -> out4/1
  demux/6 -> out5/1
  in11/1 -> mux1/6
  delayMatch/1 -> Serializer_Subnetwork1/2(in1)
  in9/1 -> mux1/5
  in7/1 -> mux1/4
  counter/1(out0) -> Serializer_Subnetwork/2(in1), delayMatch/1
  in5/1 -> mux1/3
  in3/1 -> mux1/2
  mux/1 -> Serializer_Subnetwork/1(in0)
  enb_counter_ge_7/1 -> enb_counter_ge_7_and_enb_counter_le_12/1
  in1/1 -> mux1/1
  enb_counter_le_6/1 -> counter/Enable
  in12/1 -> mux/7
  demux/3 -> out2/1
  demux/4 -> out3/1
  in10/1 -> mux/6
  in8/1 -> mux/5
  in6/1 -> mux/4
  enb_counter_le_12/1 -> enb_counter_ge_7_and_enb_counter_le_12/2
  in4/1 -> mux/3
  in2/1 -> mux/2
  in0/1 -> mux/1
  enb_counter/1 -> enb_counter_le_6/1, enb_counter_ge_7/1, enb_counter_le_12/1, enb_counter_eq_13/1

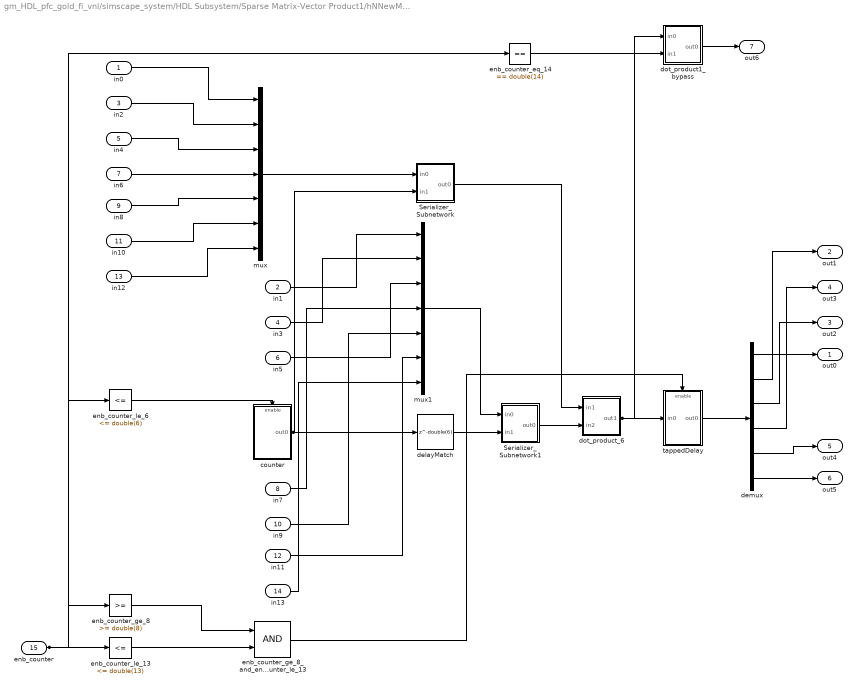
== system gm_HDL_pfc_gold_fi_vnl/simscape_system/HDL Subsystem/Sparse Matrix-Vector Product1/hNNewMatrixA_shared ==
  in0 : Inport  OutDataTypeStr=fixdt(1, 25, 24)  PortDimensions=[6]  SampleTime=1.38600138600139e-08
  in1 : Inport  Port=2  OutDataTypeStr=fixdt(1, 25, 13)  PortDimensions=[6]  SampleTime=1.38600138600139e-08
  in2 : Inport  Port=3  OutDataTypeStr=fixdt(1, 25, 24)  PortDimensions=[6]  SampleTime=1.38600138600139e-08
  in3 : Inport  Port=4  OutDataTypeStr=fixdt(1, 25, 13)  PortDimensions=[6]  SampleTime=1.38600138600139e-08
  in4 : Inport  Port=5  OutDataTypeStr=fixdt(1, 25, 24)  PortDimensions=[6]  SampleTime=1.38600138600139e-08
  in5 : Inport  Port=6  OutDataTypeStr=fixdt(1, 25, 13)  PortDimensions=[6]  SampleTime=1.38600138600139e-08
  in6 : Inport  Port=7  OutDataTypeStr=fixdt(1, 25, 24)  PortDimensions=[6]  SampleTime=1.38600138600139e-08
  in7 : Inport  Port=8  OutDataTypeStr=fixdt(1, 25, 13)  PortDimensions=[6]  SampleTime=1.38600138600139e-08
  in8 : Inport  Port=9  OutDataTypeStr=fixdt(1, 25, 24)  PortDimensions=[6]  SampleTime=1.38600138600139e-08
  in9 : Inport  Port=10  OutDataTypeStr=fixdt(1, 25, 13)  PortDimensions=[6]  SampleTime=1.38600138600139e-08
  in10 : Inport  Port=11  OutDataTypeStr=fixdt(1, 25, 24)  PortDimensions=[6]  SampleTime=1.38600138600139e-08
  in11 : Inport  Port=12  OutDataTypeStr=fixdt(1, 25, 13)  PortDimensions=[6]  SampleTime=1.38600138600139e-08
  in12 : Inport  Port=13  OutDataTypeStr=fixdt(1, 25, 24)  PortDimensions=[6]  SampleTime=1.38600138600139e-08
  in13 : Inport  Port=14  OutDataTypeStr=fixdt(1, 25, 13)  PortDimensions=[6]  SampleTime=1.38600138600139e-08
  enb_counter : Inport  Port=15  OutDataTypeStr=fixdt(0, 6, 0)  SampleTime=1.38600138600139e-08
  Serializer_Subnetwork : Subsystem
  Serializer_Subnetwork1 : Subsystem
  counter : Subsystem
  delayMatch : Delay  DelayLength=double(6)  InitialCondition=0  SampleTime=1.38600138600139e-08
  demux : Demux  Outputs=6
  dot_product1_bypass : Subsystem
  dot_product_6 : Subsystem
  enb_counter_eq_14 : simulink/Logic and Bit Operations/Compare To Constant  relop===  const=double(14)  OutDataTypeStr=boolean
  enb_counter_ge_8 : simulink/Logic and Bit Operations/Compare To Constant  relop=>=  const=double(8)  OutDataTypeStr=boolean
  enb_counter_ge_8_and_enb_counter_le_13 : Logic  AllPortsSameDT=off  OutDataTypeStr=boolean  SampleTime=1.38600138600139e-08
  enb_counter_le_13 : simulink/Logic and Bit Operations/Compare To Constant  relop=<=  const=double(13)  OutDataTypeStr=boolean
  enb_counter_le_6 : simulink/Logic and Bit Operations/Compare To Constant  relop=<=  const=double(6)  OutDataTypeStr=boolean
  mux : Mux  Inputs=7
  mux1 : Mux  Inputs=7
  tappedDelay : Subsystem
  out0 : Outport  OutDataTypeStr=fixdt(1, 50, 37)  SampleTime=1.38600138600139e-08
  out1 : Outport  Port=2  OutDataTypeStr=fixdt(1, 50, 37)  SampleTime=1.38600138600139e-08
  out2 : Outport  Port=3  OutDataTypeStr=fixdt(1, 50, 37)  SampleTime=1.38600138600139e-08
  out3 : Outport  Port=4  OutDataTypeStr=fixdt(1, 50, 37)  SampleTime=1.38600138600139e-08
  out4 : Outport  Port=5  OutDataTypeStr=fixdt(1, 50, 37)  SampleTime=1.38600138600139e-08
  out5 : Outport  Port=6  OutDataTypeStr=fixdt(1, 50, 37)  SampleTime=1.38600138600139e-08
  out6 : Outport  Port=7  OutDataTypeStr=fixdt(1, 50, 37)  SampleTime=1.38600138600139e-08
  wires:
  demux/5 -> out4/1
  demux/6 -> out5/1
  demux/3 -> out2/1
  demux/4 -> out3/1
  demux/2 -> out1/1
  dot_product1_bypass/1(out0) -> out6/1
  delayMatch/1 -> Serializer_Subnetwork1/2(in1)
  mux1/1 -> Serializer_Subnetwork1/1(in0)
  tappedDelay/1(out0) -> demux/1
  enb_counter_ge_8_and_enb_counter_le_13/1 -> tappedDelay/Enable
  in13/1 -> mux1/7
  in11/1 -> mux1/6
  in9/1 -> mux1/5
  in7/1 -> mux1/4
  counter/1(out0) -> Serializer_Subnetwork/2(in1), delayMatch/1
  dot_product_6/1(out1) -> dot_product1_bypass/1(in0), tappedDelay/1(in0)
  in5/1 -> mux1/3
  in3/1 -> mux1/2
  Serializer_Subnetwork1/1(out0) -> dot_product_6/2(in2)
  in1/1 -> mux1/1
  enb_counter_eq_14/1 -> dot_product1_bypass/2(in1)
  enb_counter_le_13/1 -> enb_counter_ge_8_and_enb_counter_le_13/2
  enb_counter_ge_8/1 -> enb_counter_ge_8_and_enb_counter_le_13/1
  enb_counter_le_6/1 -> counter/Enable
  in12/1 -> mux/7
  mux/1 -> Serializer_Subnetwork/1(in0)
  Serializer_Subnetwork/1(out0) -> dot_product_6/1(in1)
  in10/1 -> mux/6
  in8/1 -> mux/5
  in6/1 -> mux/4
  in4/1 -> mux/3
  in2/1 -> mux/2
  in0/1 -> mux/1
  demux/1 -> out0/1
  enb_counter/1 -> enb_counter_le_6/1, enb_counter_le_13/1, enb_counter_ge_8/1, enb_counter_eq_14/1

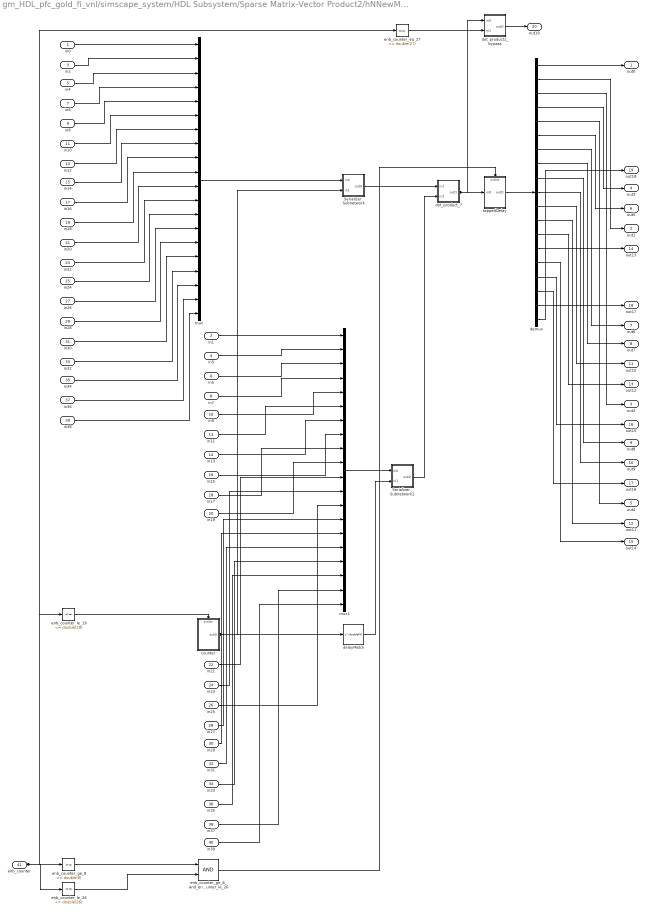
== system gm_HDL_pfc_gold_fi_vnl/simscape_system/HDL Subsystem/Sparse Matrix-Vector Product2/hNNewMatrixC_shared ==
  in0 : Inport  OutDataTypeStr=fixdt(1, 25, 20)  PortDimensions=[7]  SampleTime=1.38600138600139e-08
  in1 : Inport  Port=2  OutDataTypeStr=fixdt(1, 25, 13)  PortDimensions=[7]  SampleTime=1.38600138600139e-08
  in2 : Inport  Port=3  OutDataTypeStr=fixdt(1, 25, 20)  PortDimensions=[7]  SampleTime=1.38600138600139e-08
  in3 : Inport  Port=4  OutDataTypeStr=fixdt(1, 25, 13)  PortDimensions=[7]  SampleTime=1.38600138600139e-08
  in4 : Inport  Port=5  OutDataTypeStr=fixdt(1, 25, 20)  PortDimensions=[7]  SampleTime=1.38600138600139e-08
  in5 : Inport  Port=6  OutDataTypeStr=fixdt(1, 25, 13)  PortDimensions=[7]  SampleTime=1.38600138600139e-08
  in6 : Inport  Port=7  OutDataTypeStr=fixdt(1, 25, 20)  PortDimensions=[7]  SampleTime=1.38600138600139e-08
  in7 : Inport  Port=8  OutDataTypeStr=fixdt(1, 25, 13)  PortDimensions=[7]  SampleTime=1.38600138600139e-08
  in8 : Inport  Port=9  OutDataTypeStr=fixdt(1, 25, 20)  PortDimensions=[7]  SampleTime=1.38600138600139e-08
  in9 : Inport  Port=10  OutDataTypeStr=fixdt(1, 25, 13)  PortDimensions=[7]  SampleTime=1.38600138600139e-08
  in10 : Inport  Port=11  OutDataTypeStr=fixdt(1, 25, 20)  PortDimensions=[7]  SampleTime=1.38600138600139e-08
  in11 : Inport  Port=12  OutDataTypeStr=fixdt(1, 25, 13)  PortDimensions=[7]  SampleTime=1.38600138600139e-08
  in12 : Inport  Port=13  OutDataTypeStr=fixdt(1, 25, 20)  PortDimensions=[7]  SampleTime=1.38600138600139e-08
  in13 : Inport  Port=14  OutDataTypeStr=fixdt(1, 25, 13)  PortDimensions=[7]  SampleTime=1.38600138600139e-08
  in14 : Inport  Port=15  OutDataTypeStr=fixdt(1, 25, 20)  PortDimensions=[7]  SampleTime=1.38600138600139e-08
  in15 : Inport  Port=16  OutDataTypeStr=fixdt(1, 25, 13)  PortDimensions=[7]  SampleTime=1.38600138600139e-08
  in16 : Inport  Port=17  OutDataTypeStr=fixdt(1, 25, 20)  PortDimensions=[7]  SampleTime=1.38600138600139e-08
  in17 : Inport  Port=18  OutDataTypeStr=fixdt(1, 25, 13)  PortDimensions=[7]  SampleTime=1.38600138600139e-08
  in18 : Inport  Port=19  OutDataTypeStr=fixdt(1, 25, 20)  PortDimensions=[7]  SampleTime=1.38600138600139e-08
  in19 : Inport  Port=20  OutDataTypeStr=fixdt(1, 25, 13)  PortDimensions=[7]  SampleTime=1.38600138600139e-08
  in20 : Inport  Port=21  OutDataTypeStr=fixdt(1, 25, 20)  PortDimensions=[7]  SampleTime=1.38600138600139e-08
  in21 : Inport  Port=22  OutDataTypeStr=fixdt(1, 25, 13)  PortDimensions=[7]  SampleTime=1.38600138600139e-08
  in22 : Inport  Port=23  OutDataTypeStr=fixdt(1, 25, 20)  PortDimensions=[7]  SampleTime=1.38600138600139e-08
  in23 : Inport  Port=24  OutDataTypeStr=fixdt(1, 25, 13)  PortDimensions=[7]  SampleTime=1.38600138600139e-08
  in24 : Inport  Port=25  OutDataTypeStr=fixdt(1, 25, 20)  PortDimensions=[7]  SampleTime=1.38600138600139e-08
  in25 : Inport  Port=26  OutDataTypeStr=fixdt(1, 25, 13)  PortDimensions=[7]  SampleTime=1.38600138600139e-08
  in26 : Inport  Port=27  OutDataTypeStr=fixdt(1, 25, 20)  PortDimensions=[7]  SampleTime=1.38600138600139e-08
  in27 : Inport  Port=28  OutDataTypeStr=fixdt(1, 25, 13)  PortDimensions=[7]  SampleTime=1.38600138600139e-08
  in28 : Inport  Port=29  OutDataTypeStr=fixdt(1, 25, 20)  PortDimensions=[7]  SampleTime=1.38600138600139e-08
  in29 : Inport  Port=30  OutDataTypeStr=fixdt(1, 25, 13)  PortDimensions=[7]  SampleTime=1.38600138600139e-08
  in30 : Inport  Port=31  OutDataTypeStr=fixdt(1, 25, 20)  PortDimensions=[7]  SampleTime=1.38600138600139e-08
  in31 : Inport  Port=32  OutDataTypeStr=fixdt(1, 25, 13)  PortDimensions=[7]  SampleTime=1.38600138600139e-08
  in32 : Inport  Port=33  OutDataTypeStr=fixdt(1, 25, 20)  PortDimensions=[7]  SampleTime=1.38600138600139e-08
  in33 : Inport  Port=34  OutDataTypeStr=fixdt(1, 25, 13)  PortDimensions=[7]  SampleTime=1.38600138600139e-08
  in34 : Inport  Port=35  OutDataTypeStr=fixdt(1, 25, 20)  PortDimensions=[7]  SampleTime=1.38600138600139e-08
  in35 : Inport  Port=36  OutDataTypeStr=fixdt(1, 25, 13)  PortDimensions=[7]  SampleTime=1.38600138600139e-08
  in36 : Inport  Port=37  OutDataTypeStr=fixdt(1, 25, 20)  PortDimensions=[7]  SampleTime=1.38600138600139e-08
  in37 : Inport  Port=38  OutDataTypeStr=fixdt(1, 25, 13)  PortDimensions=[7]  SampleTime=1.38600138600139e-08
  in38 : Inport  Port=39  OutDataTypeStr=fixdt(1, 25, 20)  PortDimensions=[7]  SampleTime=1.38600138600139e-08
  in39 : Inport  Port=40  OutDataTypeStr=fixdt(1, 25, 13)  PortDimensions=[7]  SampleTime=1.38600138600139e-08
  enb_counter : Inport  Port=41  OutDataTypeStr=fixdt(0, 6, 0)  SampleTime=1.38600138600139e-08
  Serializer_Subnetwork : Subsystem
  Serializer_Subnetwork1 : Subsystem
  counter : Subsystem
  delayMatch : Delay  DelayLength=double(6)  InitialCondition=0  SampleTime=1.38600138600139e-08
  demux : Demux  Outputs=19
  dot_product1_bypass : Subsystem
  dot_product_7 : Subsystem
  enb_counter_eq_27 : simulink/Logic and Bit Operations/Compare To Constant  relop===  const=double(27)  OutDataTypeStr=boolean
  enb_counter_ge_8 : simulink/Logic and Bit Operations/Compare To Constant  relop=>=  const=double(8)  OutDataTypeStr=boolean
  enb_counter_ge_8_and_enb_counter_le_26 : Logic  AllPortsSameDT=off  OutDataTypeStr=boolean  SampleTime=1.38600138600139e-08
  enb_counter_le_19 : simulink/Logic and Bit Operations/Compare To Constant  relop=<=  const=double(19)  OutDataTypeStr=boolean
  enb_counter_le_26 : simulink/Logic and Bit Operations/Compare To Constant  relop=<=  const=double(26)  OutDataTypeStr=boolean
  mux : Mux  Inputs=20
  mux1 : Mux  Inputs=20
  tappedDelay : Subsystem
  out0 : Outport  OutDataTypeStr=fixdt(1, 50, 33)  SampleTime=1.38600138600139e-08
  out1 : Outport  Port=2  OutDataTypeStr=fixdt(1, 50, 33)  SampleTime=1.38600138600139e-08
  out2 : Outport  Port=3  OutDataTypeStr=fixdt(1, 50, 33)  SampleTime=1.38600138600139e-08
  out3 : Outport  Port=4  OutDataTypeStr=fixdt(1, 50, 33)  SampleTime=1.38600138600139e-08
  out4 : Outport  Port=5  OutDataTypeStr=fixdt(1, 50, 33)  SampleTime=1.38600138600139e-08
  out5 : Outport  Port=6  OutDataTypeStr=fixdt(1, 50, 33)  SampleTime=1.38600138600139e-08
  out6 : Outport  Port=7  OutDataTypeStr=fixdt(1, 50, 33)  SampleTime=1.38600138600139e-08
  out7 : Outport  Port=8  OutDataTypeStr=fixdt(1, 50, 33)  SampleTime=1.38600138600139e-08
  out8 : Outport  Port=9  OutDataTypeStr=fixdt(1, 50, 33)  SampleTime=1.38600138600139e-08
  out9 : Outport  Port=10  OutDataTypeStr=fixdt(1, 50, 33)  SampleTime=1.38600138600139e-08
  out10 : Outport  Port=11  OutDataTypeStr=fixdt(1, 50, 33)  SampleTime=1.38600138600139e-08
  out11 : Outport  Port=12  OutDataTypeStr=fixdt(1, 50, 33)  SampleTime=1.38600138600139e-08
  out12 : Outport  Port=13  OutDataTypeStr=fixdt(1, 50, 33)  SampleTime=1.38600138600139e-08
  out13 : Outport  Port=14  OutDataTypeStr=fixdt(1, 50, 33)  SampleTime=1.38600138600139e-08
  out14 : Outport  Port=15  OutDataTypeStr=fixdt(1, 50, 33)  SampleTime=1.38600138600139e-08
  out15 : Outport  Port=16  OutDataTypeStr=fixdt(1, 50, 33)  SampleTime=1.38600138600139e-08
  out16 : Outport  Port=17  OutDataTypeStr=fixdt(1, 50, 33)  SampleTime=1.38600138600139e-08
  out17 : Outport  Port=18  OutDataTypeStr=fixdt(1, 50, 33)  SampleTime=1.38600138600139e-08
  out18 : Outport  Port=19  OutDataTypeStr=fixdt(1, 50, 33)  SampleTime=1.38600138600139e-08
  out19 : Outport  Port=20  OutDataTypeStr=fixdt(1, 50, 33)  SampleTime=1.38600138600139e-08
  wires:
  demux/19 -> out18/1
  demux/18 -> out17/1
  demux/17 -> out16/1
  demux/16 -> out15/1
  demux/13 -> out12/1
  demux/12 -> out11/1
  demux/11 -> out10/1
  demux/10 -> out9/1
  demux/5 -> out4/1
  demux/6 -> out5/1
  mux1/1 -> Serializer_Subnetwork1/1(in0)
  dot_product1_bypass/1(out0) -> out19/1
  enb_counter_ge_8_and_enb_counter_le_26/1 -> tappedDelay/Enable
  in39/1 -> mux1/20
  in37/1 -> mux1/19
  in35/1 -> mux1/18
  in33/1 -> mux1/17
  in29/1 -> mux1/15
  in27/1 -> mux1/14
  demux/14 -> out13/1
  enb_counter_eq_27/1 -> dot_product1_bypass/2(in1)
  demux/7 -> out6/1
  demux/8 -> out7/1
  in25/1 -> mux1/13
  demux/1 -> out0/1
  demux/2 -> out1/1
  in23/1 -> mux1/12
  in19/1 -> mux1/10
  in17/1 -> mux1/9
  in15/1 -> mux1/8
  in13/1 -> mux1/7
  in11/1 -> mux1/6
  in9/1 -> mux1/5
  in7/1 -> mux1/4
  in3/1 -> mux1/2
  in1/1 -> mux1/1
  in31/1 -> mux1/16
  mux/1 -> Serializer_Subnetwork/1(in0)
  in5/1 -> mux1/3
  enb_counter_le_26/1 -> enb_counter_ge_8_and_enb_counter_le_26/2
  enb_counter_ge_8/1 -> enb_counter_ge_8_and_enb_counter_le_26/1
  in21/1 -> mux1/11
  dot_product_7/1(out1) -> dot_product1_bypass/1(in0), tappedDelay/1(in0)
  in38/1 -> mux/20
  in36/1 -> mux/19
  counter/1(out0) -> Serializer_Subnetwork/2(in1), delayMatch/1
  in34/1 -> mux/18
  delayMatch/1 -> Serializer_Subnetwork1/2(in1)
  in32/1 -> mux/17
  tappedDelay/1(out0) -> demux/1
  in30/1 -> mux/16
  in28/1 -> mux/15
  demux/15 -> out14/1
  demux/9 -> out8/1
  in26/1 -> mux/14
  demux/3 -> out2/1
  in24/1 -> mux/13
  demux/4 -> out3/1
  in22/1 -> mux/12
  in20/1 -> mux/11
  in18/1 -> mux/10
  in16/1 -> mux/9
  enb_counter_le_19/1 -> counter/Enable
  in14/1 -> mux/8
  in12/1 -> mux/7
  in10/1 -> mux/6
  Serializer_Subnetwork/1(out0) -> dot_product_7/1(in1)
  in6/1 -> mux/4
  in4/1 -> mux/3
  in2/1 -> mux/2
  in0/1 -> mux/1
  enb_counter/1 -> enb_counter_le_19/1, enb_counter_ge_8/1, enb_counter_eq_27/1, enb_counter_le_26/1
  Serializer_Subnetwork1/1(out0) -> dot_product_7/2(in2)
  in8/1 -> mux/5
